simulink model "full_state_linear_SPMSG"  (R2020b)
settings: Solver=FixedStepAuto  StartTime=0  StopTime=2  FixedStep=5e-7  RelTol=1e-3
undefined symbols (not defined in the file): capacitance, DiscIntNeverNeededParam, LdRated, LqRated, PhiPMRated, Pn, Rsnubber, RsRated, speed, TsimCurLoop, TsimMotor
libraries: powerlib x18, slpidlib x3, simulink x2, powerlib_meascontrol x2
(part 1 of 2)
settings Model: SimulationMode=accelerator  Creator=73775  LastModifiedBy=73775
settings DataIOCC: ReturnWorkspaceOutputs=off

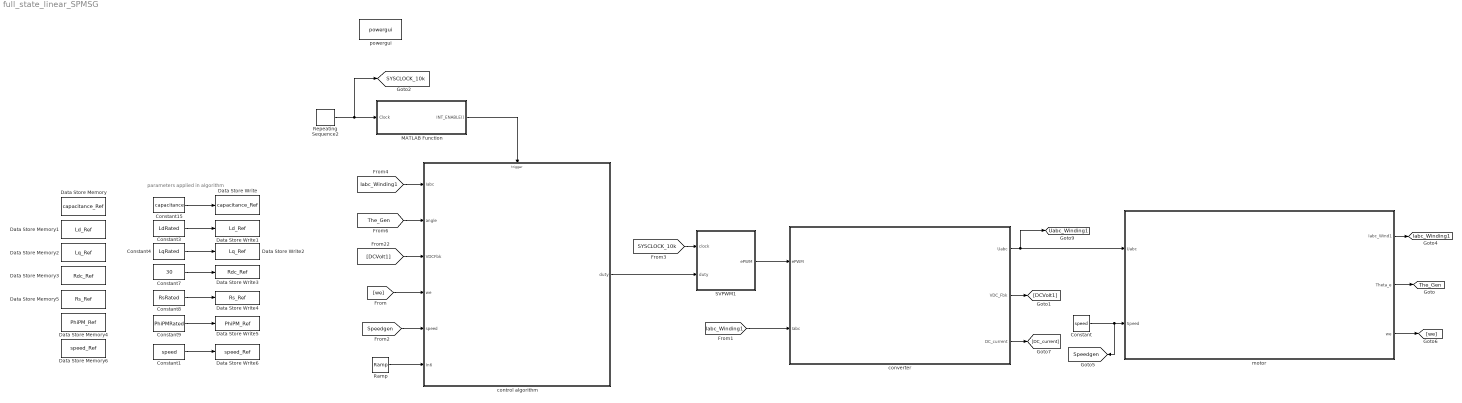
== system full_state_linear_SPMSG ==
  note: parameters applied in algorithm
  Constant : Constant  Value=speed  SampleTime=TsimMotor
  Constant1 : Constant  Value=speed  SampleTime=TsimMotor
  Constant15 : Constant  Value=capacitance  SampleTime=TsimMotor
  Constant3 : Constant  Value=LdRated  SampleTime=TsimMotor
  Constant4 : Constant  Value=LqRated  SampleTime=TsimMotor
  Constant7 : Constant  Value=30  SampleTime=TsimMotor
  Constant8 : Constant  Value=RsRated  SampleTime=TsimMotor
  Constant9 : Constant  Value=PhiPMRated  SampleTime=TsimMotor
  Data Store Memory : DataStoreMemory  DataStoreName=capacitance_Ref  ReadBeforeWriteMsg=warning  WriteAfterWriteMsg=warning  WriteAfterReadMsg=warning  ShowAdditionalParam=off
  Data Store Memory1 : DataStoreMemory  DataStoreName=Ld_Ref  ReadBeforeWriteMsg=warning  WriteAfterWriteMsg=warning  WriteAfterReadMsg=warning  ShowAdditionalParam=off
  Data Store Memory2 : DataStoreMemory  DataStoreName=Lq_Ref  ReadBeforeWriteMsg=warning  WriteAfterWriteMsg=warning  WriteAfterReadMsg=warning  ShowAdditionalParam=off
  Data Store Memory3 : DataStoreMemory  DataStoreName=Rdc_Ref  ReadBeforeWriteMsg=warning  WriteAfterWriteMsg=warning  WriteAfterReadMsg=warning  ShowAdditionalParam=off
  Data Store Memory4 : DataStoreMemory  DataStoreName=PhiPM_Ref  ReadBeforeWriteMsg=warning  WriteAfterWriteMsg=warning  WriteAfterReadMsg=warning  ShowAdditionalParam=off
  Data Store Memory5 : DataStoreMemory  DataStoreName=Rs_Ref  ReadBeforeWriteMsg=warning  WriteAfterWriteMsg=warning  WriteAfterReadMsg=warning  ShowAdditionalParam=off
  Data Store Memory6 : DataStoreMemory  DataStoreName=speed_Ref  ReadBeforeWriteMsg=warning  WriteAfterWriteMsg=warning  WriteAfterReadMsg=warning  ShowAdditionalParam=off
  Data Store Write : DataStoreWrite  DataStoreName=capacitance_Ref
  Data Store Write1 : DataStoreWrite  DataStoreName=Ld_Ref
  Data Store Write2 : DataStoreWrite  DataStoreName=Lq_Ref
  Data Store Write3 : DataStoreWrite  DataStoreName=Rdc_Ref
  Data Store Write4 : DataStoreWrite  DataStoreName=Rs_Ref
  Data Store Write5 : DataStoreWrite  DataStoreName=PhiPM_Ref
  Data Store Write6 : DataStoreWrite  DataStoreName=speed_Ref
  MATLAB Function : MATLAB Function  TreatAsAtomicUnit=on
  Ramp : simulink/Sources/Ramp  slope=1000  start=0  InitialOutput=28
  Repeating Sequence2 : simulink/Sources/Repeating Sequence  rep_seq_t=[0 0.5*TsimCurLoop 1*TsimCurLoop]  rep_seq_y=[0 1/20000 0]
  SVPWM1 : Subsystem
  control algorithm : Subsystem  TreatAsAtomicUnit=on
  converter : Subsystem
  motor : Subsystem
  powergui : powerlib/powergui  Priority=1  SimulationMode=Discrete  SampleTime=TsimMotor  frequency=60  Iterations=50  frequencyindice=0  Pbase=100e6  ErrMax=1e-4  UnitsV=kV  UnitsW=MW  buscounter=0  FunctionMessages=off  echomessages=off  EnableUseOfTLC=off  CurrentSourceSwitches=off  DisableSnubberDevices=off  DisableRonSwitches=off  DisableVfSwitches=off  DisplayEquations=off  AutomaticDiscreteSolvers=off  SolverType=Tustin/Backward Euler (TBE)  Interpol=off  ExternalGateDelay=off  methode=off  Ts=100  x0status=blocks  SPID=on  SwTol=0  HookPort=off  NonlinearTolerance=1e-4  nMaxIteration=100  ContinueOnMaxIteration=off  RestoreLinks=warning  ResistiveCurrentMeasurement=off  Frange=[0:2:500]  Ylog=off  Xlog=on  ShowGrid=off  save=off  variable=ZData  structure=Ia  ZoomFFT=off  StartTime=0.2  cycles=5  DisplayStyle=3  fundamental=67  FreqAxis=on  MaxFrequency=2000  frequencyindicesteady=1  RmsSteady=1  display=off
  tag scope: Iabc_Winding1=global, SYSCLOCK_10k=global, Speedgen=global, The_Gen=global, Uabc_Winding1=global
  wires:
  motor/2(Theta_e) -> [The_Gen]
  motor/1(Iabc_Wind1) -> [Iabc_Winding1]
  MATLAB Function/1(INT_ENABLE()) -> control algorithm/Trigger
  Repeating Sequence2/1 -> [SYSCLOCK_10k], MATLAB Function/1(Clock)
  control algorithm/1(duty) -> SVPWM1/2(duty)
  [SYSCLOCK_10k] -> SVPWM1/1(clock)
  motor/3(we) -> [we]
  [we] -> control algorithm/4(we)
  Constant/1 -> [Speedgen], motor/2("Speed ")
  [The_Gen] -> control algorithm/2(angle)
  [Speedgen] -> control algorithm/5(speed)
  converter/1(Uabc) -> [Uabc_Winding1], motor/1(Uabc)
  SVPWM1/1(ePWM) -> converter/1(ePWM)
  [Iabc_Winding1] -> converter/2(Iabc)
  converter/2(VDC_Fbk) -> [DCVolt1]
  converter/3(DC_current) -> [DC_current]
  [Iabc_Winding1] -> control algorithm/1(Iabc)
  [DCVolt1] -> control algorithm/3(VDCFbk)
  Ramp/1 -> control algorithm/6(In6)
  Constant15/1 -> Data Store Write/1
  Constant3/1 -> Data Store Write1/1
  Constant4/1 -> Data Store Write2/1
  Constant7/1 -> Data Store Write3/1
  Constant8/1 -> Data Store Write4/1
  Constant9/1 -> Data Store Write5/1
  Constant1/1 -> Data Store Write6/1

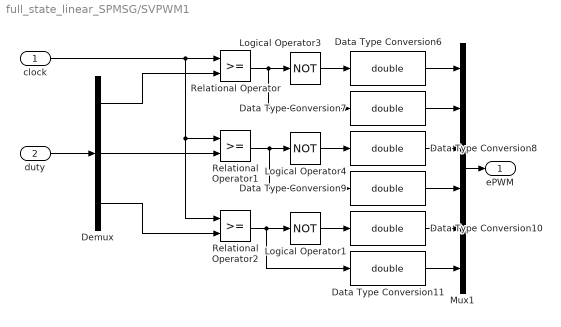
== system full_state_linear_SPMSG/SVPWM1 ==
  clock : Inport
  duty : Inport  Port=2
  Data Type Conversion{6..11} (6 alike) : DataTypeConversion  OutDataTypeStr=double
  Demux : Demux  Outputs=3
  Logical Operator1 : Logic  Operator=NOT  AllPortsSameDT=off  OutDataTypeStr=boolean
  Logical Operator3 : Logic  Operator=NOT  AllPortsSameDT=off  OutDataTypeStr=boolean
  Logical Operator4 : Logic  Operator=NOT  AllPortsSameDT=off  OutDataTypeStr=boolean
  Mux1 : Mux  Inputs=6
  Relational Operator : RelationalOperator  OutDataTypeStr=boolean  RndMeth=Simplest
  Relational Operator1 : RelationalOperator  OutDataTypeStr=boolean  RndMeth=Simplest
  Relational Operator2 : RelationalOperator  OutDataTypeStr=boolean  RndMeth=Simplest
  ePWM : Outport
  wires:
  Data Type Conversion6/1 -> Mux1/1
  Data Type Conversion11/1 -> Mux1/6
  Data Type Conversion7/1 -> Mux1/2
  Data Type Conversion10/1 -> Mux1/5
  Data Type Conversion9/1 -> Mux1/4
  Data Type Conversion8/1 -> Mux1/3
  duty/1 -> Demux/1
  Demux/3 -> Relational Operator2/2
  Mux1/1 -> ePWM/1
  Demux/2 -> Relational Operator1/2
  Relational Operator/1 -> Data Type Conversion7/1, Logical Operator3/1
  Demux/1 -> Relational Operator/2
  Relational Operator2/1 -> Data Type Conversion11/1, Logical Operator1/1
  clock/1 -> Relational Operator/1, Relational Operator1/1, Relational Operator2/1
  Relational Operator1/1 -> Data Type Conversion9/1, Logical Operator4/1
  Logical Operator3/1 -> Data Type Conversion6/1
  Logical Operator4/1 -> Data Type Conversion8/1
  Logical Operator1/1 -> Data Type Conversion10/1

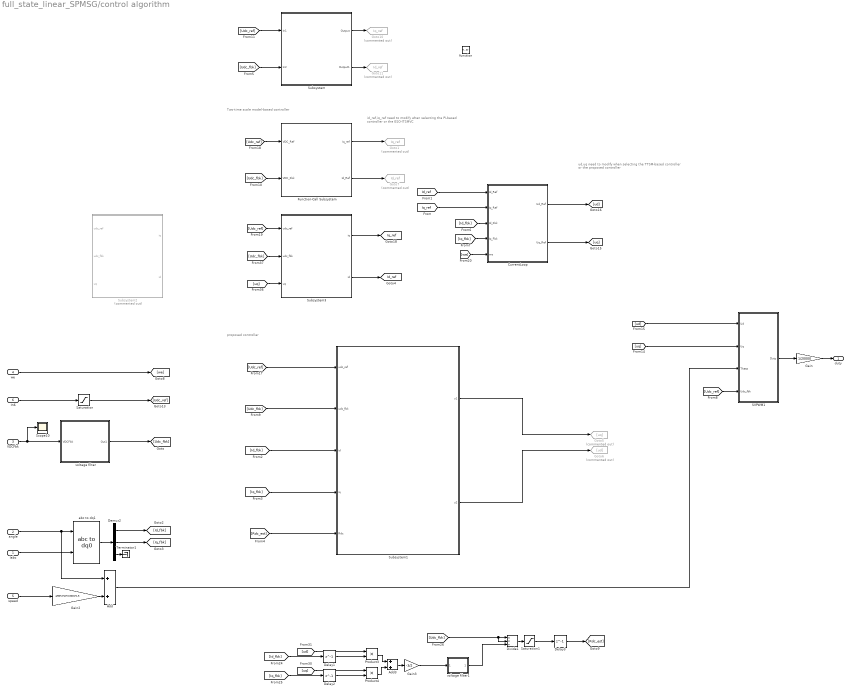
== system full_state_linear_SPMSG/control algorithm ==
  note: proposed controller
  note: Two-time scale model-based controller
  note: ud,uq
      | need to modify when selecting the TTSM-based
      | controller or the proposed controller
  note: id_ref,iq_ref
      | need to modify when selecting the PI-based
      | controller or the ESO-ITSMVC
  Iabc : Inport
  angle : Inport  Port=2
  VDCFbk : Inport  Port=3
  we : Inport  Port=4
  speed : Inport  Port=5
  In6 : Inport  Port=6
  function : TriggerPort  TriggerType=function-call  VariantControl=Variant
  Add : Sum
  Add3 : Sum
  CurrentLoop : Subsystem  mask{kp=0.075, ki=100}
      mask Display:
      | color('blue');
      | disp('current controller');
      | color('black');
      | port_label('input',1,'Id ref','texmode','on');
      | port_label('input',2,'Iq ref','texmode','on');
      | port_label('input',3,'Id fbk','texmode','on');
      | port_label('input',4,'Iq fbk','texmode','on');
      | port_label('input',5,'we','texmode','on');
      | port_label('output',1,'ud ref','texmode','on');
      | port_label('output',2,'uq ref','texmode','on');
  Delay1 : Delay  DelayLength=1
  Delay2 : Delay  DelayLength=1
  Delay3 : Delay  DelayLength=1
  Demux2 : Demux  Outputs=3
  Divide1 : Product  Inputs=**/
  Function-Call Subsystem : Subsystem  TreatAsAtomicUnit=on  mask{kp=0.03, ki=1.6}
      mask Display:
      | color('blue');
      | disp('PI-based voltage controller');
      | color('black');
      | port_label('input',1,'Udc ref','texmode','on');
      | port_label('input',2,'Udc fbk','texmode','on');
      | port_label('output',1,'Iq ref','texmode','on');
      | port_label('output',2,'Id ref','texmode','on');
  Gain : Gain  Gain=1/20000
  Gain2 : Gain  Gain=4/60*2*pi*0.0001*1.5
  Gain3 : Gain  Gain=-3/2
  Goto1 : Goto  Commented=on  GotoTag=Iq_ref  TagVisibility=global
  Goto10 : Goto  Commented=on  GotoTag=Iq_ref  TagVisibility=global
  Goto11 : Goto  Commented=on  GotoTag=Id_ref  TagVisibility=global
  Goto5 : Goto  Commented=on  GotoTag=uq
  Goto6 : Goto  Commented=on  GotoTag=ud
  Goto7 : Goto  Commented=on  GotoTag=Id_ref  TagVisibility=global
  Product3 : Product
  Product4 : Product
  SVPWM1 : Subsystem
  Saturation : Saturate  UpperLimit=48  LowerLimit=0
  Saturation1 : Saturate  UpperLimit=100  LowerLimit=10
  Scope10 : Scope
  Subsystem : Subsystem  mask{k=0.06, n=1e-3}
      mask Display:
      | color('blue');
      | disp('adaptive voltage controller');
      | color('black');
      | port_label('input',1,'Udc ref','texmode','on');
      | port_label('input',2,'Udc fbk','texmode','on');
      | port_label('output',1,'Iq ref','texmode','on');
      | port_label('output',2,'Id ref','texmode','on');
  Subsystem1 : Subsystem  mask{k0=235000000, k1=11990000, k2=5000, k3=800, k4=160000, k5=0.15}
      mask Display:
      | color('blue');
      | disp('proposed integrated controller');
      | color('black');
      | port_label('input',1,'Udc ref','texmode','on');
      | port_label('input',2,'Udc fbk','texmode','on');
      | port_label('input',3,'Id fbk','texmode','on');
      | port_label('input',4,'Iq fbk','texmode','on');
      | port_label('output',1,'uq','texmode','on');
      | port_label('output',2,'ud','texmode','on');
  Subsystem2 : Subsystem  Commented=on  mask{c=0.1, r=0.017, n=0.02, b1=170, b2=14500}
      mask prompts: c "intergrel term in s"; r "product term of s"; n "product term of sgn(s)"; b1 "b1 in ESO"; b2 "b2 in ESO"
      mask Display:
      | color('blue');
      | disp('ESO-ITSMVC');
      | color('black');
      | port_label('input',1,'Udc ref','texmode','on');
      | port_label('input',2,'Udc fbk','texmode','on');
      | port_label('input',3,'uq','texmode','on');
      | port_label('output',1,'Iq ref','texmode','on');
      | port_label('output',2,'Id ref','texmode','on');
  Subsystem3 : Subsystem  mask{c=250, r=0.06, n=0.02, b1=3000, b2=2250000}
      mask prompts: c "intergrel term in s"; r "product term of s"; n "product term of sgn(s)"; b1 "b1 in ESO"; b2 "b2 in ESO"
      mask Display:
      | color('blue');
      | disp('ESO-ITSMVC');
      | color('black');
      | port_label('input',1,'Udc ref','texmode','on');
      | port_label('input',2,'Udc fbk','texmode','on');
      | port_label('input',3,'uq','texmode','on');
      | port_label('output',1,'Iq ref','texmode','on');
      | port_label('output',2,'Id ref','texmode','on');
  Terminator1 : Terminator
  abc to dq1 : powerlib_meascontrol/Transformations/abc to dq0  Alignment=Aligned with phase A axis
  voltage filter : Subsystem
  voltage filter1 : Subsystem
  duty : Outport
  tag scope: Id_ref=global, Iq_ref=global
  wires:
  Iabc/1 -> abc to dq1/1
  abc to dq1/1 -> Demux2/1
  Demux2/3 -> Terminator1/1
  [Id_ref] -> CurrentLoop/1(Id_Ref)
  [Iq_ref] -> CurrentLoop/2(Iq_Ref)
  Demux2/1 -> [Id_fbk]
  Demux2/2 -> [Iq_fbk]
  we/1 -> [we]
  SVPWM1/1(Duty) -> Gain/1
  Gain/1 -> duty/1
  VDCFbk/1 -> voltage filter/1(VDCFbk), Scope10/1
  Add/1 -> SVPWM1/3(Theta)
  speed/1 -> Gain2/1
  Gain2/1 -> Add/2
  [Udc_ref] -> SVPWM1/4(Udc_fbk)
  CurrentLoop/1(Ud_Ref) -> [ud]
  CurrentLoop/2(Uq_Ref) -> [uq]
  angle/1 -> Add/1, abc to dq1/2
  [ud] -> SVPWM1/1(Ud)
  [uq] -> SVPWM1/2(Uq)
  [Udc_ref] -> Function-Call Subsystem/1(VDC_Ref)
  [Udc_fbk] -> Function-Call Subsystem/2(VDC_Fbk)
  In6/1 -> Saturation/1
  [uq] -> Subsystem3/3(uq)
  [Id_fbk] -> CurrentLoop/3(Id_Fbk)
  [Iq_fbk] -> CurrentLoop/4(Iq_Fbk)
  Saturation/1 -> [Udc_ref]
  Subsystem3/1(iq) -> [Iq_ref]
  Subsystem3/2(id) -> [Id_ref]
  [Udc_ref] -> Subsystem3/1(udc_ref)
  [Udc_fbk] -> Subsystem3/2(udc_fbk)
  [we] -> CurrentLoop/5(we)
  [Udc_ref] -> Subsystem1/1(udc_ref)
  [Udc_fbk] -> Subsystem1/2(udc_fbk)
  Subsystem1/1(u1) -> Goto5/1
  Subsystem1/2(u2) -> Goto6/1
  [Id_fbk] -> Subsystem1/3(id)
  [Iq_fbk] -> Subsystem1/4(iq)
  Function-Call Subsystem/2(Id_Ref) -> Goto7/1
  voltage filter/1(Out1) -> [Udc_fbk]
  Product3/1 -> Add3/1
  Add3/1 -> Gain3/1
  [ud] -> Product3/1
  Delay1/1 -> Product3/2
  Divide1/1 -> Saturation1/1
  [uq] -> Product4/1
  Product4/1 -> Add3/2
  [Udc_fbk] -> Divide1/1, Divide1/2
  [Id_fbk] -> Delay1/1
  Delay2/1 -> Product4/2
  [Iq_fbk] -> Delay2/1
  [Rdc_est] -> Subsystem1/5(Rdc)
  Saturation1/1 -> Delay3/1
  Gain3/1 -> voltage filter1/1(VDCFbk)
  voltage filter1/1(Out1) -> Divide1/3
  Delay3/1 -> [Rdc_est]
  [Udc_ref] -> Subsystem/1(In1)
  [Udc_fbk] -> Subsystem/2(In2)
  Subsystem/1(Output) -> Goto10/1
  Subsystem/2(Output1) -> Goto11/1
  Function-Call Subsystem/1(Iq_ref) -> Goto1/1

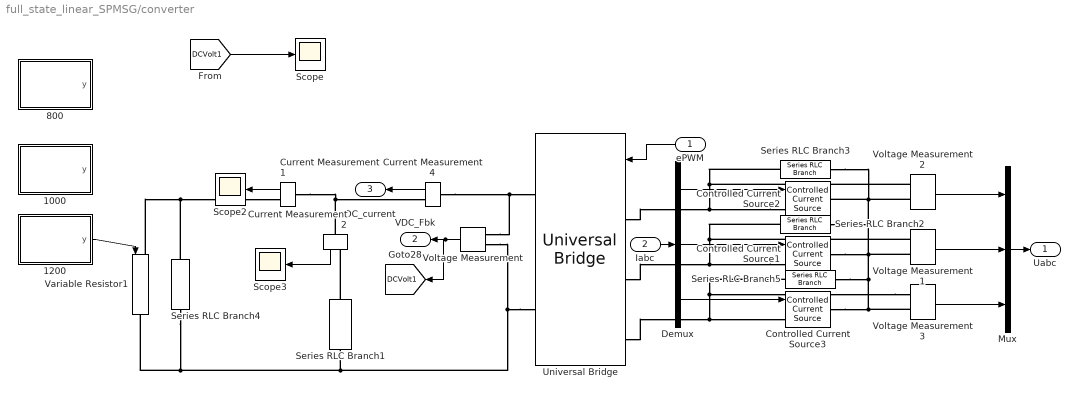
== system full_state_linear_SPMSG/converter ==
  ePWM : Inport
  Iabc : Inport  Port=2
  1000 : MATLAB Function  TreatAsAtomicUnit=on
  1200 : MATLAB Function  TreatAsAtomicUnit=on
  800 : MATLAB Function  TreatAsAtomicUnit=on
  Controlled Current Source1 : powerlib/Electrical Sources/Controlled Current Source  Initialize=on  Source_Type=AC  Amplitude=0  Phase=0  Frequency=0  Measurements=None
  Controlled Current Source2 : powerlib/Electrical Sources/Controlled Current Source  Initialize=on  Source_Type=AC  Amplitude=0  Phase=0  Frequency=0  Measurements=None
  Controlled Current Source3 : powerlib/Electrical Sources/Controlled Current Source  Initialize=on  Source_Type=AC  Amplitude=0  Phase=0  Frequency=0  Measurements=None
  Current Measurement1 : powerlib/Measurements/Current Measurement  PhasorSimulation=off  OutputType=Complex  PSBequivalent=0
  Current Measurement2 : powerlib/Measurements/Current Measurement  PhasorSimulation=off  OutputType=Complex  PSBequivalent=0
  Current Measurement4 : powerlib/Measurements/Current Measurement  PhasorSimulation=off  OutputType=Complex  PSBequivalent=0
  Demux : Demux  Outputs=3
  Mux : Mux  Inputs=3
  Scope : Scope
  Scope2 : Scope
  Scope3 : Scope
  Series RLC Branch1 : powerlib/Elements/Series RLC Branch  LConnTagsString=__new0  RConnTagsString=__new0  BranchType=C  Resistance=1  Inductance=51.869e-9  SetiL0=off  InitialCurrent=0  Capacitance=capacitance  Setx0=on  InitialVoltage=28  Measurements=None
  Series RLC Branch2 : powerlib/Elements/Series RLC Branch  LConnTagsString=__new0  RConnTagsString=__new0  BranchType=R  Resistance=Rsnubber  Inductance=51.869e-9  SetiL0=off  InitialCurrent=0  Capacitance=330e-6  Setx0=off  InitialVoltage=0  Measurements=None
  Series RLC Branch3 : powerlib/Elements/Series RLC Branch  LConnTagsString=__new0  RConnTagsString=__new0  BranchType=R  Resistance=Rsnubber  Inductance=51.869e-9  SetiL0=off  InitialCurrent=0  Capacitance=330e-6  Setx0=off  InitialVoltage=0  Measurements=None
  Series RLC Branch4 : powerlib/Elements/Series RLC Branch  LConnTagsString=__new0  RConnTagsString=__new0  BranchType=R  Resistance=100  Inductance=51.869e-9  SetiL0=off  InitialCurrent=0  Capacitance=330e-6  Setx0=off  InitialVoltage=0  Measurements=None
  Series RLC Branch5 : powerlib/Elements/Series RLC Branch  LConnTagsString=__new0  RConnTagsString=__new0  BranchType=R  Resistance=Rsnubber  Inductance=51.869e-9  SetiL0=off  InitialCurrent=0  Capacitance=330e-6  Setx0=off  InitialVoltage=0  Measurements=None
  Universal Bridge : powerlib/Power Electronics/Universal Bridge  Arms=3  SnubberResistance=Rsnubber  SnubberCapacitance=inf  Device=IGBT / Diodes  Ron=0.02  Lon=0  ForwardVoltages="[  0  0  ]"  ForwardVoltage=0  GTOparameters=[ 10e-6 , 20e-6 ]  IGBTparameters=[ 1e-6 , 2e-6 ]  Measurements=None  Measurements_2=None  converterType=Rectifier
  Variable Resistor1 : powerlib/Elements/Variable Resistor  Rabsmin=1e-3
      settings: SourceProductBaseCode=PS
  Voltage Measurement{,1..3} (4 alike) : powerlib/Measurements/Voltage Measurement  PhasorSimulation=off  OutputType=Complex  PSBequivalent=0
  Uabc : Outport
  VDC_Fbk : Outport  Port=2
  DC_current : Outport  Port=3
  tag scope: DCVolt1=global
  wires:
  Voltage Measurement/1 -> [DCVolt1], VDC_Fbk/1
  Demux/1 -> Controlled Current Source2/1
  Demux/3 -> Controlled Current Source3/1
  Voltage Measurement1/1 -> Mux/2
  Voltage Measurement2/1 -> Mux/1
  Demux/2 -> Controlled Current Source1/1
  Voltage Measurement3/1 -> Mux/3
  Mux/1 -> Uabc/1
  ePWM/1 -> Universal Bridge/1
  Iabc/1 -> Demux/1
  Current Measurement4/1 -> DC_current/1
  Current Measurement1/1 -> Scope2/1
  Current Measurement2/1 -> Scope3/1
  [DCVolt1] -> Scope/1
  1200/1(y) -> Variable Resistor1/1
  connections:
  Universal Bridge/RConn2 -- Series RLC Branch4/RConn1 -- Variable Resistor1/RConn1 -- Series RLC Branch1/RConn1 -- Voltage Measurement/LConn2
  Voltage Measurement2/LConn2 -- Controlled Current Source2/RConn1 -- Controlled Current Source1/RConn1 -- Voltage Measurement1/LConn2 -- Voltage Measurement3/LConn2 -- Controlled Current Source3/RConn1 -- Series RLC Branch5/RConn1 -- Series RLC Branch2/RConn1 -- Series RLC Branch3/RConn1
  Voltage Measurement/LConn1 -- Current Measurement4/LConn1 -- Universal Bridge/RConn1
  Controlled Current Source2/LConn1 -- Universal Bridge/LConn1 -- Voltage Measurement2/LConn1 -- Series RLC Branch3/LConn1
  Voltage Measurement3/LConn1 -- Controlled Current Source3/LConn1 -- Universal Bridge/LConn3 -- Series RLC Branch5/LConn1
  Controlled Current Source1/LConn1 -- Universal Bridge/LConn2 -- Series RLC Branch2/LConn1 -- Voltage Measurement1/LConn1
  Current Measurement1/LConn1 -- Current Measurement2/LConn1 -- Current Measurement4/RConn1
  Variable Resistor1/LConn1 -- Series RLC Branch4/LConn1 -- Current Measurement1/RConn1
  Series RLC Branch1/LConn1 -- Current Measurement2/RConn1

== system full_state_linear_SPMSG/motor ==
  Uabc : Inport
  "Speed " : Inport  Port=2
  Add : Sum  Inputs=+-
  Clark Transformation : Subsystem
  Demux : Demux  Outputs=3
  Electrical Model Simplied1 : Subsystem
  "Mechanical Model " : Subsystem
  Mux1 : Mux  Inputs=3
  Park Transformation : Subsystem
  VSINonlinearity : Subsystem
  dq0 to abc1 : powerlib_meascontrol/Transformations/dq0 to abc  Alignment=Aligned with phase A axis
  Iabc_Wind1 : Outport
  Theta_e : Outport  Port=2
  we : Outport  Port=3
  wires:
  Clark Transformation/1(Alpha) -> Park Transformation/1(Alpha)
  Clark Transformation/2(Beta) -> Park Transformation/2(Beta)
  "Mechanical Model "/1(Theta_e) -> Park Transformation/3(theta), Theta_e/1, dq0 to abc1/2
  Demux/1 -> Clark Transformation/1(U)
  Demux/2 -> Clark Transformation/2(V)
  Demux/3 -> Clark Transformation/3(W)
  Mux1/1 -> dq0 to abc1/1
  "Mechanical Model "/2(we) -> Electrical Model Simplied1/3(we), we/1
  "Speed "/1 -> "Mechanical Model "/1(speed)
  dq0 to abc1/1 -> VSINonlinearity/1(IABC), Iabc_Wind1/1
  Park Transformation/1(D) -> Electrical Model Simplied1/1(Ud)
  Park Transformation/2(Q) -> Electrical Model Simplied1/2(Uq)
  Electrical Model Simplied1/1(Id) -> Mux1/1
  Electrical Model Simplied1/2(Iq) -> Mux1/2
  Add/1 -> Demux/1
  Uabc/1 -> Add/1
  VSINonlinearity/1(UError) -> Add/2

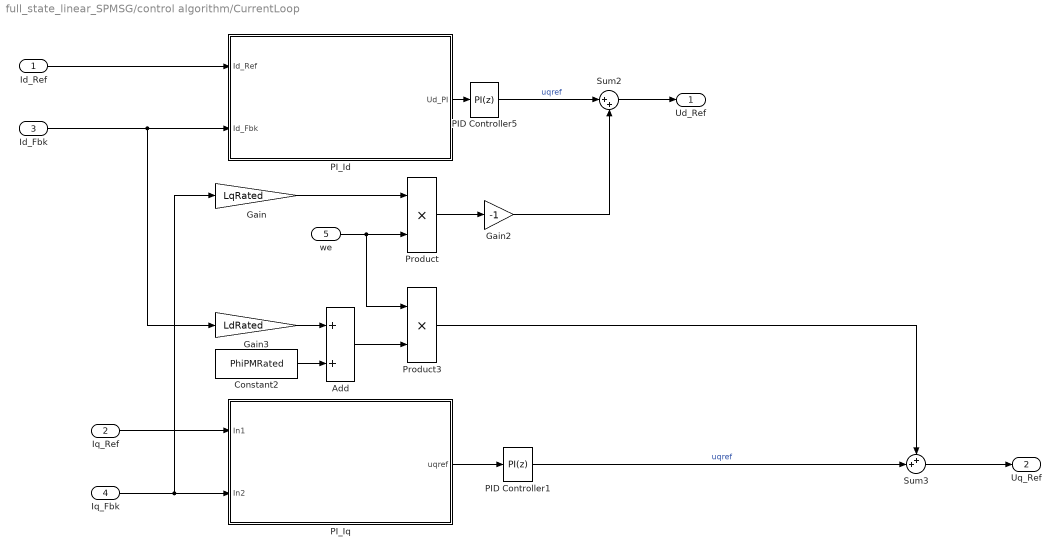
== system full_state_linear_SPMSG/control algorithm/CurrentLoop ==
  Id_Ref : Inport
  Iq_Ref : Inport  Port=2
  Id_Fbk : Inport  Port=3
  Iq_Fbk : Inport  Port=4
  we : Inport  Port=5
  Add : Sum
  Constant2 : Constant  Value=PhiPMRated  SampleTime=-1
  Gain : Gain  Gain=LqRated
  Gain2 : Gain  Gain=-1
  Gain3 : Gain  Gain=LdRated
  PID Controller1 : slpidlib/PID Controller  Controller=PI  Form=Parallel  TimeDomain=Discrete-time  UseExternalTs=off  SampleTime=-1  IntegratorMethod=Forward Euler  FilterMethod=Forward Euler  ControllerParametersSource=internal  P=kp  I=ki  D=0  UseFilter=on  N=100  TunerSelectOption=Transfer Function Based (PID Tuner App)  InitialConditionSource=internal  InitialConditionForIntegrator=0  InitialConditionForFilter=0  DifferentiatorICPrevScaledInput=0  ExternalReset=none  TrackingMode=off  Kt=1  LimitOutput=on  SatLimitsSource=internal  UpperSaturationLimit=800  LowerSaturationLimit=-800  LinearizeAsGain=on  AntiWindupMode=none  Kb=1  POutMin=[]  POutMax=[]  IOutMin=[]  IOutMax=[]  DOutMin=[]  DOutMax=[]  NOutMin=[]  NOutMax=[]  SumOutMin=-800  SumOutMax=800  SaturationOutMin=-800  SaturationOutMax=800  PParamMin=[]  PParamMax=[]  IParamMin=[]  IParamMax=[]  DParamMin=[]  DParamMax=[]  NParamMin=[]  NParamMax=[]  KbParamMin=[]  KbParamMax=[]  KtParamMin=[]  KtParamMax=[]  KbOutMin=[]  KbOutMax=[]  KtOutMin=[]  KtOutMax=[]  IntegratorOutMin=[]  IntegratorOutMax=[]  FilterOutMin=[]  FilterOutMax=[]  SumI1OutMin=[]  SumI1OutMax=[]  SumI2OutMin=[]  SumI2OutMax=[]  SumI3OutMin=[]  SumI3OutMax=[]  SumI4OutMin=[]  SumI4OutMax=[]  SumDOutMin=[]  SumDOutMax=[]  DifferentiatorOutMin=[]  DifferentiatorOutMax=[]  FilterDiffOutCoefMin=[]  FilterDiffOutCoefMax=[]  ReciprocalOutMin=[]  ReciprocalOutMax=[]  SumDenOutMin=[]  SumDenOutMax=[]  SumNumOutMin=[]  SumNumOutMax=[]  DivideOutMin=[]  DivideOutMax=[]  UdiffTsProdOutMin=[]  UdiffTsProdOutMax=[]  NTsProdOutMin=[]  NTsProdOutMax=[]  UintegralTsProdOutMin=[]  UintegralTsProdOutMax=[]  UngainTsProdOutMin=[]  UngainTsProdOutMax=[]  IntegratorContinuousStateAttributes=''  IntegratorStateMustResolveToSignalObject=off  IntegratorRTWStateStorageClass=Auto  FilterContinuousStateAttributes=''  FilterStateMustResolveToSignalObject=off  FilterRTWStateStorageClass=Auto  ParallelPVariant=InternalParameters  IdealPVariant=Disabled  IVariant=InternalParameters  DVariant=Disabled  IntegratorVariant=Discrete  SatVariant=Enabled  AWVariant=Passthrough  PCopyVariant=Disabled  TRVariant=Disabled  FdbkBlocksVariant=Forward  IdealPFdbkVariant=Disabled  SatFdbkVariant=Disabled  DerivativeFilterVariant=Disabled  NVariant=Disabled  NCopyVariant=Disabled_SignalSpec  FilterICVariant=Disabled  IntegratorICVariant=InternalICs  ExternalResetVariant=Disabled  TRSumVariant=Passthrough  SumFdbkVariant=Disabled  SumVariant=Sum_PI  TsampFilterVariant=InternalTs  TsampNgainVariant=Passthrough  TsampIntegralVariant=Passthrough  ExternalSaturationOutDataTypeStr=Inherit: Same as second input
  PID Controller5 : slpidlib/PID Controller  Controller=PI  Form=Parallel  TimeDomain=Discrete-time  UseExternalTs=off  SampleTime=-1  IntegratorMethod=Forward Euler  FilterMethod=Forward Euler  ControllerParametersSource=internal  P=kp  I=ki  D=0  UseFilter=on  N=100  TunerSelectOption=Transfer Function Based (PID Tuner App)  InitialConditionSource=internal  InitialConditionForIntegrator=0  InitialConditionForFilter=0  DifferentiatorICPrevScaledInput=0  ExternalReset=none  TrackingMode=off  Kt=1  LimitOutput=on  SatLimitsSource=internal  UpperSaturationLimit=800  LowerSaturationLimit=-800  LinearizeAsGain=on  AntiWindupMode=none  Kb=1  POutMin=[]  POutMax=[]  IOutMin=[]  IOutMax=[]  DOutMin=[]  DOutMax=[]  NOutMin=[]  NOutMax=[]  SumOutMin=-800  SumOutMax=800  SaturationOutMin=-800  SaturationOutMax=800  PParamMin=[]  PParamMax=[]  IParamMin=[]  IParamMax=[]  DParamMin=[]  DParamMax=[]  NParamMin=[]  NParamMax=[]  KbParamMin=[]  KbParamMax=[]  KtParamMin=[]  KtParamMax=[]  KbOutMin=[]  KbOutMax=[]  KtOutMin=[]  KtOutMax=[]  IntegratorOutMin=[]  IntegratorOutMax=[]  FilterOutMin=[]  FilterOutMax=[]  SumI1OutMin=[]  SumI1OutMax=[]  SumI2OutMin=[]  SumI2OutMax=[]  SumI3OutMin=[]  SumI3OutMax=[]  SumI4OutMin=[]  SumI4OutMax=[]  SumDOutMin=[]  SumDOutMax=[]  DifferentiatorOutMin=[]  DifferentiatorOutMax=[]  FilterDiffOutCoefMin=[]  FilterDiffOutCoefMax=[]  ReciprocalOutMin=[]  ReciprocalOutMax=[]  SumDenOutMin=[]  SumDenOutMax=[]  SumNumOutMin=[]  SumNumOutMax=[]  DivideOutMin=[]  DivideOutMax=[]  UdiffTsProdOutMin=[]  UdiffTsProdOutMax=[]  NTsProdOutMin=[]  NTsProdOutMax=[]  UintegralTsProdOutMin=[]  UintegralTsProdOutMax=[]  UngainTsProdOutMin=[]  UngainTsProdOutMax=[]  IntegratorContinuousStateAttributes=''  IntegratorStateMustResolveToSignalObject=off  IntegratorRTWStateStorageClass=Auto  FilterContinuousStateAttributes=''  FilterStateMustResolveToSignalObject=off  FilterRTWStateStorageClass=Auto  ParallelPVariant=InternalParameters  IdealPVariant=Disabled  IVariant=InternalParameters  DVariant=Disabled  IntegratorVariant=Discrete  SatVariant=Enabled  AWVariant=Passthrough  PCopyVariant=Disabled  TRVariant=Disabled  FdbkBlocksVariant=Forward  IdealPFdbkVariant=Disabled  SatFdbkVariant=Disabled  DerivativeFilterVariant=Disabled  NVariant=Disabled  NCopyVariant=Disabled_SignalSpec  FilterICVariant=Disabled  IntegratorICVariant=InternalICs  ExternalResetVariant=Disabled  TRSumVariant=Passthrough  SumFdbkVariant=Disabled  SumVariant=Sum_PI  TsampFilterVariant=InternalTs  TsampNgainVariant=Passthrough  TsampIntegralVariant=Passthrough  ExternalSaturationOutDataTypeStr=Inherit: Same as second input
  PI_Id : Subsystem
  PI_Iq : Subsystem
  Product : Product
  Product3 : Product
  Sum2 : Sum  Inputs=|++
  Sum3 : Sum  Inputs=++|
  Ud_Ref : Outport
  Uq_Ref : Outport  Port=2
  wires:
  Id_Fbk/1 -> PI_Id/2(Id_Fbk), Gain3/1
  Iq_Ref/1 -> PI_Iq/1(In1)
  Gain/1 -> Product/1
  Gain3/1 -> Add/1
  Constant2/1 -> Add/2
  Add/1 -> Product3/2
  we/1 -> Product3/1, Product/2
  Iq_Fbk/1 -> Gain/1, PI_Iq/2(In2)
  PI_Id/1(Ud_PI) -> PID Controller5/1
  PI_Iq/1(uqref) -> PID Controller1/1
  Product/1 -> Gain2/1
  Sum2/1 -> Ud_Ref/1
  Gain2/1 -> Sum2/2
  Sum3/1 -> Uq_Ref/1
  PID Controller1/1 -> Sum3/2  "uqref"
  Id_Ref/1 -> PI_Id/1(Id_Ref)
  PID Controller5/1 -> Sum2/1  "uqref"
  Product3/1 -> Sum3/1

== system full_state_linear_SPMSG/control algorithm/Function-Call Subsystem ==
  VDC_Ref : Inport
  VDC_Fbk : Inport  Port=2
  Add3 : Sum  Inputs=|+-
  Constant : Constant  Value=0  SampleTime=-1
  Gain : Gain  Gain=-1
  PID Controller1 : slpidlib/PID Controller  Controller=PI  Form=Parallel  TimeDomain=Discrete-time  UseExternalTs=off  SampleTime=-1  IntegratorMethod=Forward Euler  FilterMethod=Forward Euler  ControllerParametersSource=internal  P=kp  I=ki  D=0  UseFilter=on  N=100  TunerSelectOption=Transfer Function Based (PID Tuner App)  InitialConditionSource=internal  InitialConditionForIntegrator=0  InitialConditionForFilter=0  DifferentiatorICPrevScaledInput=0  ExternalReset=none  TrackingMode=off  Kt=1  LimitOutput=off  SatLimitsSource=internal  UpperSaturationLimit=640000  LowerSaturationLimit=-640000  LinearizeAsGain=on  AntiWindupMode=none  Kb=1  POutMin=[]  POutMax=[]  IOutMin=[]  IOutMax=[]  DOutMin=[]  DOutMax=[]  NOutMin=[]  NOutMax=[]  SumOutMin=-800  SumOutMax=800  SaturationOutMin=-800  SaturationOutMax=800  PParamMin=[]  PParamMax=[]  IParamMin=[]  IParamMax=[]  DParamMin=[]  DParamMax=[]  NParamMin=[]  NParamMax=[]  KbParamMin=[]  KbParamMax=[]  KtParamMin=[]  KtParamMax=[]  KbOutMin=[]  KbOutMax=[]  KtOutMin=[]  KtOutMax=[]  IntegratorOutMin=[]  IntegratorOutMax=[]  FilterOutMin=[]  FilterOutMax=[]  SumI1OutMin=[]  SumI1OutMax=[]  SumI2OutMin=[]  SumI2OutMax=[]  SumI3OutMin=[]  SumI3OutMax=[]  SumI4OutMin=[]  SumI4OutMax=[]  SumDOutMin=[]  SumDOutMax=[]  DifferentiatorOutMin=[]  DifferentiatorOutMax=[]  FilterDiffOutCoefMin=[]  FilterDiffOutCoefMax=[]  ReciprocalOutMin=[]  ReciprocalOutMax=[]  SumDenOutMin=[]  SumDenOutMax=[]  SumNumOutMin=[]  SumNumOutMax=[]  DivideOutMin=[]  DivideOutMax=[]  UdiffTsProdOutMin=[]  UdiffTsProdOutMax=[]  NTsProdOutMin=[]  NTsProdOutMax=[]  UintegralTsProdOutMin=[]  UintegralTsProdOutMax=[]  UngainTsProdOutMin=[]  UngainTsProdOutMax=[]  IntegratorContinuousStateAttributes=''  IntegratorStateMustResolveToSignalObject=off  IntegratorRTWStateStorageClass=Auto  FilterContinuousStateAttributes=''  FilterStateMustResolveToSignalObject=off  FilterRTWStateStorageClass=Auto  ParallelPVariant=InternalParameters  IdealPVariant=Disabled  IVariant=InternalParameters  DVariant=Disabled  IntegratorVariant=Discrete  SatVariant=Disabled  AWVariant=Passthrough  PCopyVariant=Disabled  TRVariant=Disabled  FdbkBlocksVariant=Forward  IdealPFdbkVariant=Disabled  SatFdbkVariant=Disabled  DerivativeFilterVariant=Disabled  NVariant=Disabled  NCopyVariant=Disabled_SignalSpec  FilterICVariant=Disabled  IntegratorICVariant=InternalICs  ExternalResetVariant=Disabled  TRSumVariant=Passthrough  SumFdbkVariant=Disabled  SumVariant=Sum_PI  TsampFilterVariant=InternalTs  TsampNgainVariant=Passthrough  TsampIntegralVariant=Passthrough  ExternalSaturationOutDataTypeStr=Inherit: Same as second input
  Product : Product
  Product1 : Product
  Iq_ref : Outport
  Id_Ref : Outport  Port=2
  wires:
  Add3/1 -> PID Controller1/1
  Constant/1 -> Id_Ref/1
  PID Controller1/1 -> Gain/1
  Gain/1 -> Iq_ref/1
  Product/1 -> Add3/1
  VDC_Ref/1 -> Product/1, Product/2
  VDC_Fbk/1 -> Product1/2, Product1/1
  Product1/1 -> Add3/2

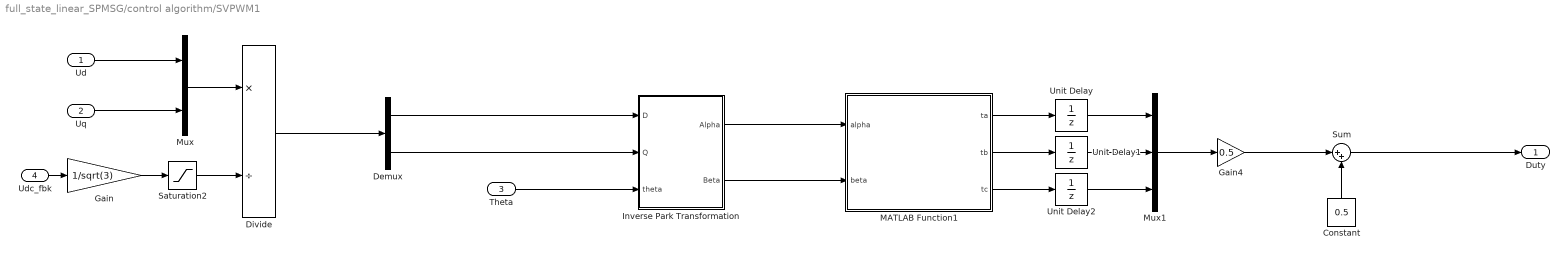
== system full_state_linear_SPMSG/control algorithm/SVPWM1 ==
  Ud : Inport
  Uq : Inport  Port=2
  Theta : Inport  Port=3
  Udc_fbk : Inport  Port=4
  Constant : Constant  Value=0.5  SampleTime=-1
  Demux : Demux  Outputs=2
  Divide : Product  Inputs=*/
  Gain : Gain  Gain=1/sqrt(3)
  Gain4 : Gain  Gain=0.5
  Inverse Park Transformation : Subsystem
  MATLAB Function1 : MATLAB Function  TreatAsAtomicUnit=on
  Mux : Mux  Inputs=2
  Mux1 : Mux  Inputs=3
  Saturation2 : Saturate  UpperLimit=800  LowerLimit=10
  Sum : Sum  Inputs=|++
  Unit Delay : UnitDelay  SampleTime=-1  HasFrameUpgradeWarning=on
  Unit Delay1 : UnitDelay  SampleTime=-1  HasFrameUpgradeWarning=on
  Unit Delay2 : UnitDelay  SampleTime=-1  HasFrameUpgradeWarning=on
  Duty : Outport
  wires:
  Inverse Park Transformation/2(Beta) -> MATLAB Function1/2(beta)
  Divide/1 -> Demux/1
  MATLAB Function1/2(tb) -> Unit Delay1/1
  Mux/1 -> Divide/1
  Saturation2/1 -> Divide/2
  Gain/1 -> Saturation2/1
  Unit Delay1/1 -> Mux1/2
  Inverse Park Transformation/1(Alpha) -> MATLAB Function1/1(alpha)
  Unit Delay2/1 -> Mux1/3
  Theta/1 -> Inverse Park Transformation/3(theta)
  MATLAB Function1/1(ta) -> Unit Delay/1
  MATLAB Function1/3(tc) -> Unit Delay2/1
  Demux/2 -> Inverse Park Transformation/2(Q)
  Demux/1 -> Inverse Park Transformation/1(D)
  Unit Delay/1 -> Mux1/1
  Constant/1 -> Sum/2
  Gain4/1 -> Sum/1
  Mux1/1 -> Gain4/1
  Ud/1 -> Mux/1
  Uq/1 -> Mux/2
  Sum/1 -> Duty/1
  Udc_fbk/1 -> Gain/1

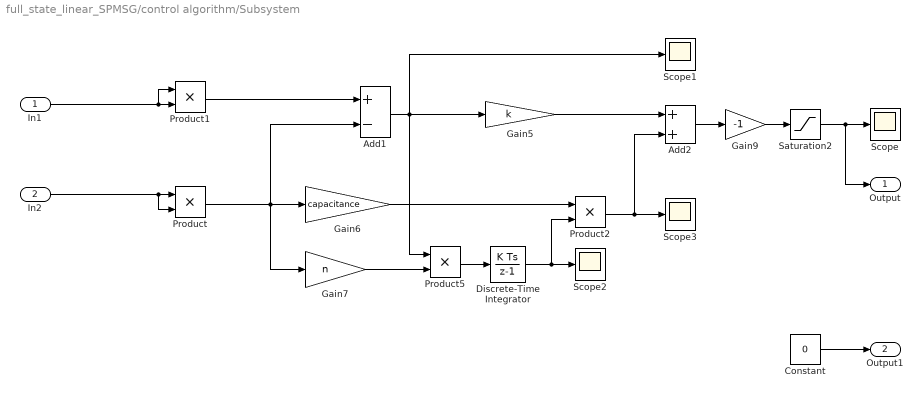
== system full_state_linear_SPMSG/control algorithm/Subsystem ==
  In1 : Inport
  In2 : Inport  Port=2
  Add1 : Sum  Inputs=+-
  Add2 : Sum
  Constant : Constant  Value=0
  Discrete-Time Integrator : DiscreteIntegrator  gainval=1  SampleTime=-1  ICPrevOutput=DiscIntNeverNeededParam  ICPrevScaledInput=DiscIntNeverNeededParam
  Gain5 : Gain  Gain=k
  Gain6 : Gain  Gain=capacitance
  Gain7 : Gain  Gain=n
  Gain9 : Gain  Gain=-1
  Product{,1..2,5} (4 alike) : Product
  Saturation2 : Saturate  UpperLimit=20  LowerLimit=-20
  Scope{,1..3} (4 alike) : Scope
  Output : Outport
  Output1 : Outport  Port=2
  wires:
  Product5/1 -> Discrete-Time Integrator/1
  In2/1 -> Product/2, Product/1
  Add1/1 -> Gain5/1, Scope1/1, Product5/1
  Discrete-Time Integrator/1 -> Product2/2, Scope2/1
  Gain5/1 -> Add2/1
  Gain6/1 -> Product2/1
  Product1/1 -> Add1/1
  Saturation2/1 -> Output/1, Scope/1
  Gain7/1 -> Product5/2
  In1/1 -> Product1/1, Product1/2
  Add2/1 -> Gain9/1
  Product2/1 -> Add2/2, Scope3/1
  Product/1 -> Gain7/1, Add1/2, Gain6/1
  Gain9/1 -> Saturation2/1
  Constant/1 -> Output1/1

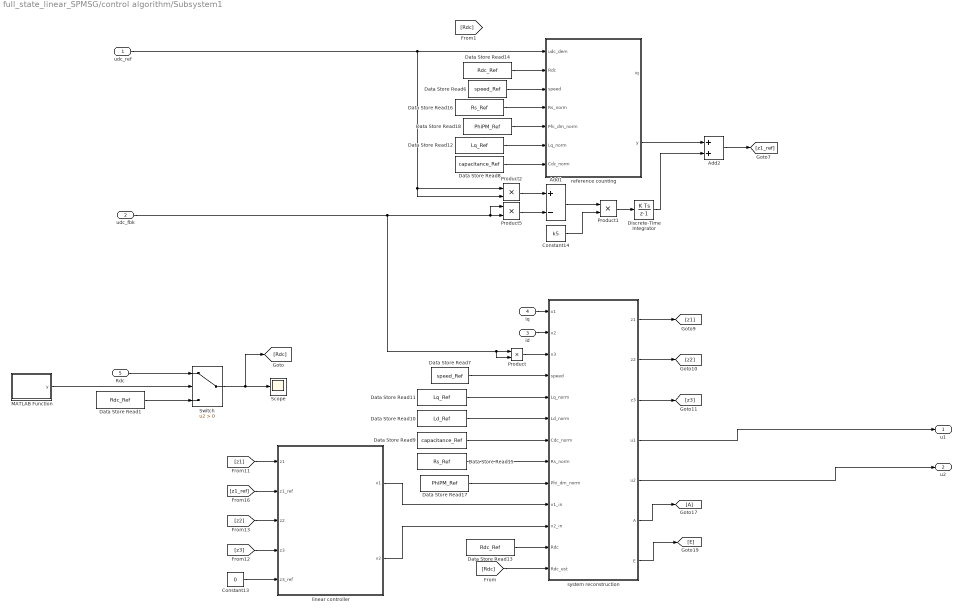
== system full_state_linear_SPMSG/control algorithm/Subsystem1 ==
  udc_ref : Inport
  udc_fbk : Inport  Port=2
  id : Inport  Port=3
  iq : Inport  Port=4
  Rdc : Inport  Port=5
  Add1 : Sum  Inputs=+-
  Add2 : Sum
  Constant13 : Constant  Value=0  SampleTime=-1
  Constant14 : Constant  Value=k5  SampleTime=-1
  Data Store Read1 : DataStoreRead  DataStoreName=Rdc_Ref
  Data Store Read10 : DataStoreRead  DataStoreName=Ld_Ref
  Data Store Read11 : DataStoreRead  DataStoreName=Lq_Ref
  Data Store Read12 : DataStoreRead  DataStoreName=Lq_Ref
  Data Store Read13 : DataStoreRead  DataStoreName=Rdc_Ref
  Data Store Read14 : DataStoreRead  DataStoreName=Rdc_Ref
  Data Store Read15 : DataStoreRead  DataStoreName=Rs_Ref
  Data Store Read16 : DataStoreRead  DataStoreName=Rs_Ref
  Data Store Read17 : DataStoreRead  DataStoreName=PhiPM_Ref
  Data Store Read18 : DataStoreRead  DataStoreName=PhiPM_Ref
  Data Store Read6 : DataStoreRead  DataStoreName=speed_Ref
  Data Store Read7 : DataStoreRead  DataStoreName=speed_Ref
  Data Store Read8 : DataStoreRead  DataStoreName=capacitance_Ref
  Data Store Read9 : DataStoreRead  DataStoreName=capacitance_Ref
  Discrete-Time Integrator : DiscreteIntegrator  SampleTime=-1  ICPrevOutput=DiscIntNeverNeededParam  ICPrevScaledInput=DiscIntNeverNeededParam
  MATLAB Function : MATLAB Function  TreatAsAtomicUnit=on
  Product{,1..2,5} (4 alike) : Product
  Scope : Scope
  Switch : Switch  Criteria=u2 > Threshold
  linear controller : Subsystem
  reference counting : MATLAB Function  TreatAsAtomicUnit=on
  system reconstruction : MATLAB Function  TreatAsAtomicUnit=on
  u1 : Outport
  u2 : Outport  Port=2
  wires:
  Data Store Read11/1 -> system reconstruction/5(Lq_norm)
  [z1] -> linear controller/1(z1)
  system reconstruction/1(z1) -> [z1]
  Data Store Read6/1 -> reference counting/3(speed)
  Data Store Read16/1 -> reference counting/4(Rs_norm)
  Data Store Read8/1 -> reference counting/7(Cdc_norm)
  Data Store Read18/1 -> reference counting/5(Phi_dm_norm)
  Product2/1 -> Add1/1
  [z3] -> linear controller/4(z3)
  Product1/1 -> Discrete-Time Integrator/1
  [z1_ref] -> linear controller/2(z1_ref)
  system reconstruction/7(E) -> [E]
  udc_fbk/1 -> Product/2, Product/1, Product5/1, Product5/2
  system reconstruction/6(A) -> [A]
  Product/1 -> system reconstruction/3(x3)
  Add1/1 -> Product1/1
  Data Store Read7/1 -> system reconstruction/4(speed)
  Constant14/1 -> Product1/2
  Data Store Read9/1 -> system reconstruction/7(Cdc_norm)
  system reconstruction/3(z3) -> [z3]
  Data Store Read15/1 -> system reconstruction/8(Rs_norm)
  linear controller/2(v2) -> system reconstruction/11(v2_in)
  Data Store Read10/1 -> system reconstruction/6(Ld_norm)
  Constant13/1 -> linear controller/5(z3_ref)
  reference counting/2(y) -> Add2/1
  Product5/1 -> Add1/2
  Discrete-Time Integrator/1 -> Add2/2
  linear controller/1(v1) -> system reconstruction/10(v1_in)
  Add2/1 -> [z1_ref]
  Data Store Read12/1 -> reference counting/6(Lq_norm)
  Data Store Read17/1 -> system reconstruction/9(Phi_dm_norm)
  system reconstruction/5(u2) -> u2/1
  system reconstruction/4(u1) -> u1/1
  udc_ref/1 -> Product2/2, Product2/1, reference counting/1(udc_dem)
  id/1 -> system reconstruction/2(x2)
  iq/1 -> system reconstruction/1(x1)
  [z2] -> linear controller/3(z2)
  Switch/1 -> [Rdc], Scope/1
  Data Store Read1/1 -> Switch/3
  Data Store Read14/1 -> reference counting/2(Rdc)
  Data Store Read13/1 -> system reconstruction/12(Rdc)
  [Rdc] -> system reconstruction/13(Rdc_est)
  system reconstruction/2(z2) -> [z2]
  Rdc/1 -> Switch/1
  MATLAB Function/1(y) -> Switch/2

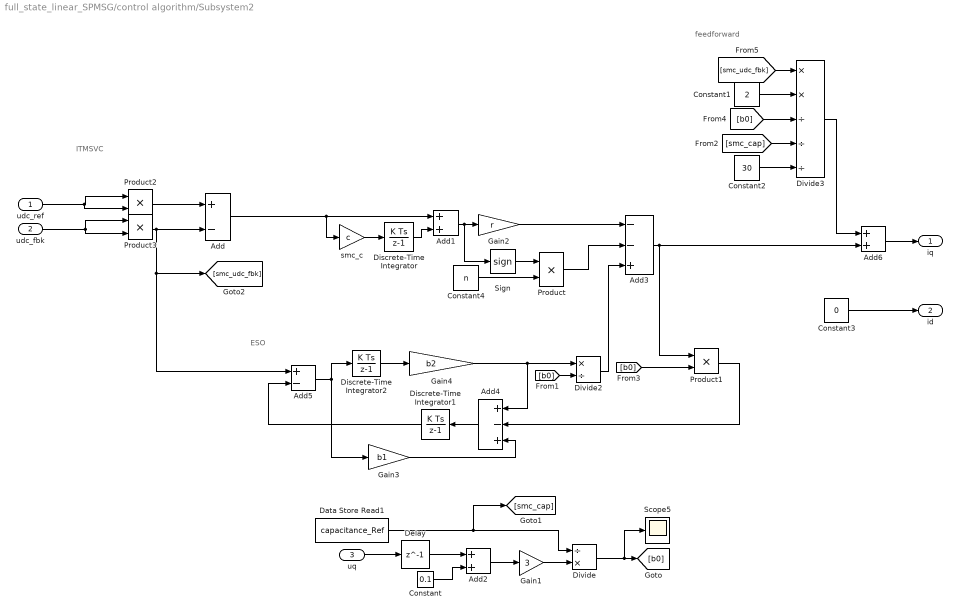
== system full_state_linear_SPMSG/control algorithm/Subsystem2 ==
  note: ESO
  note: feedforward
  note: ITMSVC
  udc_ref : Inport
  udc_fbk : Inport  Port=2
  uq : Inport  Port=3
  Add : Sum  Inputs=+-
  Add1 : Sum
  Add2 : Sum
  Add3 : Sum  Inputs=--+
  Add4 : Sum  Inputs=+-+
  Add5 : Sum  Inputs=+-
  Add6 : Sum
  Constant : Constant  Value=0.1  SampleTime=-1
  Constant1 : Constant  Value=2  SampleTime=-1
  Constant2 : Constant  Value=30  SampleTime=-1
  Constant3 : Constant  Value=0  SampleTime=-1
  Constant4 : Constant  Value=n  SampleTime=-1
  Data Store Read1 : DataStoreRead  DataStoreName=capacitance_Ref
  Delay : Delay  DelayLength=1
  Discrete-Time Integrator : DiscreteIntegrator  SampleTime=-1  ICPrevOutput=DiscIntNeverNeededParam  ICPrevScaledInput=DiscIntNeverNeededParam
  Discrete-Time Integrator1 : DiscreteIntegrator  InitialCondition=2304  SampleTime=-1  ICPrevOutput=DiscIntNeverNeededParam  ICPrevScaledInput=DiscIntNeverNeededParam
  Discrete-Time Integrator2 : DiscreteIntegrator  SampleTime=-1  ICPrevOutput=DiscIntNeverNeededParam  ICPrevScaledInput=DiscIntNeverNeededParam
  Divide : Product  Inputs=/*
  Divide2 : Product  Inputs=*/
  Divide3 : Product  Inputs=**///
  Gain1 : Gain  Gain=3
  Gain2 : Gain  Gain=r
  Gain3 : Gain  Gain=b1
  Gain4 : Gain  Gain=b2
  Product{,1..3} (4 alike) : Product
  Scope5 : Scope
  Sign : Signum
  smc_c : Gain  Gain=c
  iq : Outport
  id : Outport  Port=2
  wires:
  uq/1 -> Delay/1
  Delay/1 -> Add2/1
  udc_fbk/1 -> Product3/2, Product3/1
  Product3/1 -> Add/2, [smc_udc_fbk], Add5/1
  udc_ref/1 -> Product2/1, Product2/2
  Product2/1 -> Add/1
  Constant3/1 -> id/1
  [smc_udc_fbk] -> Divide3/1
  Product/1 -> Add3/2
  Gain2/1 -> Add3/1
  Constant4/1 -> Product/2
  Divide3/1 -> Add6/1
  Add3/1 -> Product1/1, Add6/2
  Add6/1 -> iq/1
  Divide2/1 -> Add3/3
  Constant2/1 -> Divide3/5
  [smc_cap] -> Divide3/4
  [b0] -> Divide3/3
  Constant1/1 -> Divide3/2
  Constant/1 -> Add2/2
  Discrete-Time Integrator2/1 -> Gain4/1
  Gain3/1 -> Add4/3
  Add5/1 -> Discrete-Time Integrator2/1, Gain3/1
  Discrete-Time Integrator1/1 -> Add5/2
  Add4/1 -> Discrete-Time Integrator1/1
  Product1/1 -> Add4/2
  [b0] -> Product1/2
  Gain4/1 -> Divide2/1, Add4/1
  [b0] -> Divide2/2
  Sign/1 -> Product/1
  Add1/1 -> Sign/1, Gain2/1
  Divide/1 -> [b0], Scope5/1
  Data Store Read1/1 -> Divide/1, [smc_cap]
  Gain1/1 -> Divide/2
  Add2/1 -> Gain1/1
  Discrete-Time Integrator/1 -> Add1/2
  smc_c/1 -> Discrete-Time Integrator/1
  Add/1 -> Add1/1, smc_c/1

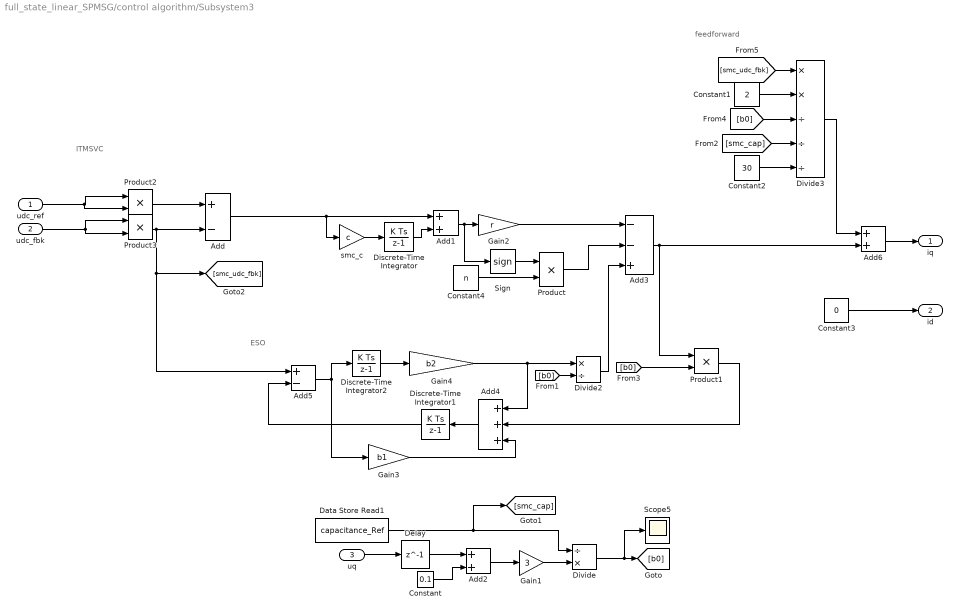
== system full_state_linear_SPMSG/control algorithm/Subsystem3 ==
  note: ITMSVC
  note: feedforward
  note: ESO
  udc_ref : Inport
  udc_fbk : Inport  Port=2
  uq : Inport  Port=3
  Add : Sum  Inputs=+-
  Add1 : Sum
  Add2 : Sum
  Add3 : Sum  Inputs=--+
  Add4 : Sum  Inputs=+++
  Add5 : Sum  Inputs=+-
  Add6 : Sum
  Constant : Constant  Value=0.1  SampleTime=-1
  Constant1 : Constant  Value=2  SampleTime=-1
  Constant2 : Constant  Value=30  SampleTime=-1
  Constant3 : Constant  Value=0  SampleTime=-1
  Constant4 : Constant  Value=n  SampleTime=-1
  Data Store Read1 : DataStoreRead  DataStoreName=capacitance_Ref
  Delay : Delay  DelayLength=1
  Discrete-Time Integrator : DiscreteIntegrator  SampleTime=-1  ICPrevOutput=DiscIntNeverNeededParam  ICPrevScaledInput=DiscIntNeverNeededParam
  Discrete-Time Integrator1 : DiscreteIntegrator  InitialCondition=2304  SampleTime=-1  ICPrevOutput=DiscIntNeverNeededParam  ICPrevScaledInput=DiscIntNeverNeededParam
  Discrete-Time Integrator2 : DiscreteIntegrator  SampleTime=-1  ICPrevOutput=DiscIntNeverNeededParam  ICPrevScaledInput=DiscIntNeverNeededParam
  Divide : Product  Inputs=/*
  Divide2 : Product  Inputs=*/
  Divide3 : Product  Inputs=**///
  Gain1 : Gain  Gain=3
  Gain2 : Gain  Gain=r
  Gain3 : Gain  Gain=b1
  Gain4 : Gain  Gain=b2
  Product{,1..3} (4 alike) : Product
  Scope5 : Scope
  Sign : Signum
  smc_c : Gain  Gain=c
  iq : Outport
  id : Outport  Port=2
  wires:
  Add/1 -> smc_c/1, Add1/1
  smc_c/1 -> Discrete-Time Integrator/1
  Discrete-Time Integrator/1 -> Add1/2
  Add2/1 -> Gain1/1
  Gain1/1 -> Divide/2
  Data Store Read1/1 -> [smc_cap], Divide/1
  Divide/1 -> Scope5/1, [b0]
  Add1/1 -> Gain2/1, Sign/1
  Sign/1 -> Product/1
  [b0] -> Divide2/2
  Gain4/1 -> Add4/1, Divide2/1
  [b0] -> Product1/2
  Product1/1 -> Add4/2
  Add4/1 -> Discrete-Time Integrator1/1
  Discrete-Time Integrator1/1 -> Add5/2
  Add5/1 -> Gain3/1, Discrete-Time Integrator2/1
  Gain3/1 -> Add4/3
  Discrete-Time Integrator2/1 -> Gain4/1
  Constant/1 -> Add2/2
  Constant1/1 -> Divide3/2
  [b0] -> Divide3/3
  [smc_cap] -> Divide3/4
  Constant2/1 -> Divide3/5
  Divide2/1 -> Add3/3
  Add6/1 -> iq/1
  Add3/1 -> Add6/2, Product1/1
  Divide3/1 -> Add6/1
  Constant4/1 -> Product/2
  Gain2/1 -> Add3/1
  Product/1 -> Add3/2
  [smc_udc_fbk] -> Divide3/1
  Constant3/1 -> id/1
  Product2/1 -> Add/1
  udc_ref/1 -> Product2/2, Product2/1
  Product3/1 -> Add5/1, [smc_udc_fbk], Add/2
  udc_fbk/1 -> Product3/1, Product3/2
  Delay/1 -> Add2/1
  uq/1 -> Delay/1

== system full_state_linear_SPMSG/control algorithm/voltage filter ==
  VDCFbk : Inport
  Add : Sum
  Add1 : Sum  Inputs=+-
  Constant : Constant  Value=1000  SampleTime=-1
  Constant1 : Constant  SampleTime=-1
  Delay : Delay  DelayLength=1
  Gain : Gain  Gain=2*pi*TsimCurLoop
  Gain1 : Gain  Gain=2*pi*TsimCurLoop
  Product : Product
  Product1 : Product
  Out1 : Outport
  wires:
  Constant/1 -> Gain1/1, Gain/1
  Gain/1 -> Product/2
  VDCFbk/1 -> Product/1
  Product/1 -> Add/1
  Add/1 -> Delay/1, Out1/1
  Delay/1 -> Product1/1
  Constant1/1 -> Add1/1
  Add1/1 -> Product1/2
  Gain1/1 -> Add1/2
  Product1/1 -> Add/2

== system full_state_linear_SPMSG/control algorithm/voltage filter1 ==
  VDCFbk : Inport
  Add : Sum
  Add1 : Sum  Inputs=+-
  Constant : Constant  Value=0.1  SampleTime=-1
  Constant1 : Constant  SampleTime=-1
  Delay : Delay  DelayLength=1
  Product : Product
  Product1 : Product
  Out1 : Outport
  wires:
  Constant/1 -> Add1/2, Product/2
  VDCFbk/1 -> Product/1
  Product/1 -> Add/1
  Constant1/1 -> Add1/1
  Add1/1 -> Product1/2
  Product1/1 -> Add/2
  [last] -> Delay/1
  Add/1 -> [last], Out1/1
  Delay/1 -> Product1/1

== system full_state_linear_SPMSG/motor/Clark Transformation ==
  U : Inport
  V : Inport  Port=2
  W : Inport  Port=3
  Add : Sum  Inputs=+--
  Add1 : Sum  Inputs=+-
  Gain : Gain  Gain=0.5
  Gain1 : Gain  Gain=0.5
  Gain2 : Gain  Gain=2/3
  Gain3 : Gain  Gain=2/3*0.86602540
  Alpha : Outport
  Beta : Outport  Port=2
  wires:
  V/1 -> Add1/1, Gain/1
  Gain/1 -> Add/2
  W/1 -> Add1/2, Gain1/1
  Gain1/1 -> Add/3
  U/1 -> Add/1
  Add/1 -> Gain2/1
  Gain2/1 -> Alpha/1
  Add1/1 -> Gain3/1
  Gain3/1 -> Beta/1

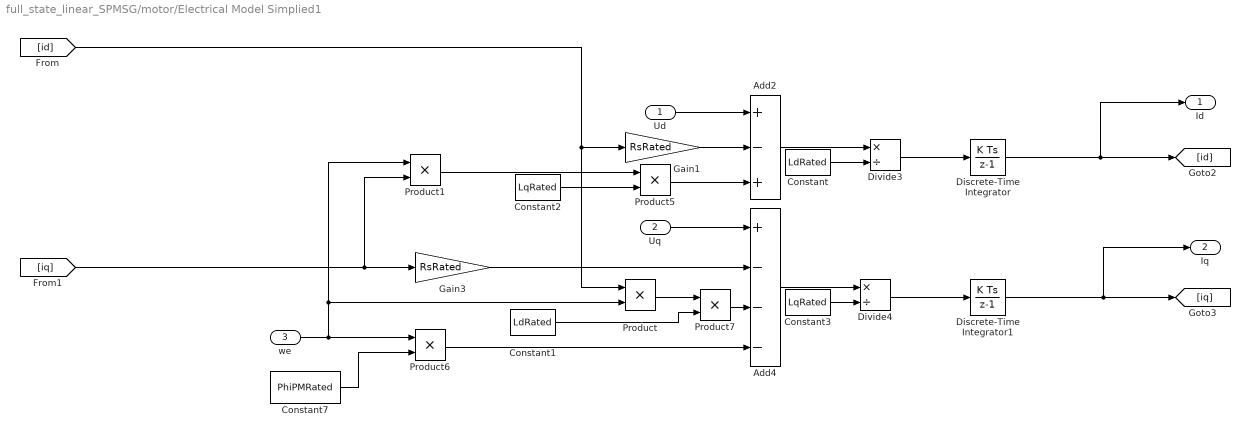
== system full_state_linear_SPMSG/motor/Electrical Model Simplied1 ==
  Ud : Inport
  Uq : Inport  Port=2
  we : Inport  Port=3
  Add2 : Sum  Inputs=+-+
  Add4 : Sum  Inputs=+---
  Constant : Constant  Value=LdRated  SampleTime=TsimMotor
  Constant1 : Constant  Value=LdRated  SampleTime=TsimMotor
  Constant2 : Constant  Value=LqRated  SampleTime=TsimMotor
  Constant3 : Constant  Value=LqRated  SampleTime=TsimMotor
  Constant7 : Constant  Value=PhiPMRated  SampleTime=TsimMotor
  Discrete-Time Integrator : DiscreteIntegrator  SampleTime=TsimMotor  ICPrevOutput=DiscIntNeverNeededParam  ICPrevScaledInput=DiscIntNeverNeededParam
  Discrete-Time Integrator1 : DiscreteIntegrator  SampleTime=TsimMotor  ICPrevOutput=DiscIntNeverNeededParam  ICPrevScaledInput=DiscIntNeverNeededParam
  Divide3 : Product  Inputs=*/
  Divide4 : Product  Inputs=*/
  Gain1 : Gain  Gain=RsRated
  Gain3 : Gain  Gain=RsRated
  Product{,1,5..7} (5 alike) : Product
  Id : Outport
  Iq : Outport  Port=2
  wires:
  Product/1 -> Product7/1
  Discrete-Time Integrator1/1 -> Iq/1, [iq]
  Product5/1 -> Add2/3
  Gain3/1 -> Add4/2
  Product6/1 -> Add4/4
  Discrete-Time Integrator/1 -> Id/1, [id]
  Product7/1 -> Add4/3
  Gain1/1 -> Add2/2
  Add4/1 -> Divide4/1
  Add2/1 -> Divide3/1
  Constant1/1 -> Product7/2
  Divide4/1 -> Discrete-Time Integrator1/1
  Divide3/1 -> Discrete-Time Integrator/1
  [id] -> Product/1, Gain1/1
  [iq] -> Product1/2, Gain3/1
  Ud/1 -> Add2/1
  Uq/1 -> Add4/1
  we/1 -> Product/2, Product1/1, Product6/1
  Constant2/1 -> Product5/2
  Constant/1 -> Divide3/2
  Constant3/1 -> Divide4/2
  Product1/1 -> Product5/1
  Constant7/1 -> Product6/2

== system full_state_linear_SPMSG/motor/Mechanical Model  ==
  speed : Inport
  Discrete-Time Integrator3 : DiscreteIntegrator  SampleTime=TsimMotor  ICPrevOutput=DiscIntNeverNeededParam  ICPrevScaledInput=DiscIntNeverNeededParam
  Gain5 : Gain  Gain=pi*Pn/30
  Theta_e : Outport
  we : Outport  Port=2
  wires:
  Discrete-Time Integrator3/1 -> [theta_e], Theta_e/1
  Gain5/1 -> we/1, Discrete-Time Integrator3/1
  speed/1 -> Gain5/1

== system full_state_linear_SPMSG/motor/Park Transformation ==
  Alpha : Inport
  Beta : Inport  Port=2
  theta : Inport  Port=3
  Add : Sum
  Add1 : Sum  Inputs=+-
  Product{,1..3} (4 alike) : Product
  Sin : Trigonometry  OutputSignalType=real
  Sin1 : Trigonometry  Operator=cos  OutputSignalType=real
  D : Outport
  Q : Outport  Port=2
  wires:
  Product/1 -> Add/1
  Sin/1 -> Product3/2, Product1/2
  Product1/1 -> Add/2
  Add1/1 -> Q/1
  Sin1/1 -> Product2/2, Product/2
  Product2/1 -> Add1/1
  Alpha/1 -> Product3/1, Product/1
  Beta/1 -> Product2/1, Product1/1
  Product3/1 -> Add1/2
  Add/1 -> D/1
  theta/1 -> Sin/1, Sin1/1

== system full_state_linear_SPMSG/motor/VSINonlinearity ==
  IABC : Inport
  Constant : Constant  Value=0.17  SampleTime=TsimMotor
  Constant1 : Constant  SampleTime=TsimMotor
  Demux1 : Demux  Outputs=3
  MATLAB Function1 : MATLAB Function  TreatAsAtomicUnit=on
  MATLAB Function2 : MATLAB Function  TreatAsAtomicUnit=on
  MATLAB Function3 : MATLAB Function  TreatAsAtomicUnit=on
  Mux1 : Mux  Inputs=3
  Scope : Scope
  UError : Outport
  wires:
  Demux1/3 -> MATLAB Function3/1(I)
  Constant1/1 -> MATLAB Function3/3(Vdead), MATLAB Function2/3(Vdead), MATLAB Function1/3(Vdead)
  Constant/1 -> MATLAB Function3/2(K), MATLAB Function2/2(K), MATLAB Function1/2(K)
  MATLAB Function3/1(U) -> Mux1/3
  Demux1/2 -> MATLAB Function2/1(I)
  MATLAB Function2/1(U) -> Mux1/2
  Demux1/1 -> MATLAB Function1/1(I)
  Mux1/1 -> UError/1
  IABC/1 -> Demux1/1
  MATLAB Function1/1(U) -> Scope/1, Mux1/1

== system full_state_linear_SPMSG/control algorithm/CurrentLoop/PI_Id ==
  Id_Ref : Inport
  Id_Fbk : Inport  Port=2
  Add1 : Sum  Inputs=|+-
  Zero-Order Hold5 : ZeroOrderHold  SampleTime=-1
  id实际值 : Scope  NumInputPorts=2
  Ud_PI : Outport
  wires:
  Zero-Order Hold5/1 -> id实际值/2, Add1/2
  Add1/1 -> Ud_PI/1  "uqref"
  Id_Fbk/1 -> Zero-Order Hold5/1
  Id_Ref/1 -> id实际值/1, Add1/1

== system full_state_linear_SPMSG/control algorithm/CurrentLoop/PI_Iq ==
  In1 : Inport
  In2 : Inport  Port=2
  Add2 : Sum  Inputs=|+-
  Zero-Order Hold1 : ZeroOrderHold  SampleTime=-1
  iq实际值 : Scope  NumInputPorts=2
  uqref : Outport
  wires:
  In1/1 -> iq实际值/1, Add2/1
  Zero-Order Hold1/1 -> iq实际值/2, Add2/2
  In2/1 -> Zero-Order Hold1/1
  Add2/1 -> uqref/1  "uqref"

== system full_state_linear_SPMSG/control algorithm/SVPWM1/Inverse Park Transformation ==
  D : Inport
  Q : Inport  Port=2
  theta : Inport  Port=3
  Product{,1..3} (4 alike) : Product  OutDataTypeStr=Inherit: Same as first input
  Sin : Trigonometry  OutputSignalType=real
  Sin1 : Trigonometry  Operator=cos  OutputSignalType=real
  Sum1 : Sum  Inputs=|++  OutDataTypeStr=Inherit: Same as first input
  Sum2 : Sum  Inputs=|+-  OutDataTypeStr=Inherit: Same as first input
  Alpha : Outport
  Beta : Outport  Port=2
  wires:
  Sin1/1 -> Product2/2, Product/2
  Sin/1 -> Product3/2, Product1/2
  Product3/1 -> Sum1/2
  Sum1/1 -> Beta/1
  D/1 -> Product3/1, Product/1
  Product2/1 -> Sum1/1
  Sum2/1 -> Alpha/1
  Product/1 -> Sum2/1
  Product1/1 -> Sum2/2
  Q/1 -> Product2/1, Product1/1
  theta/1 -> Sin/1, Sin1/1

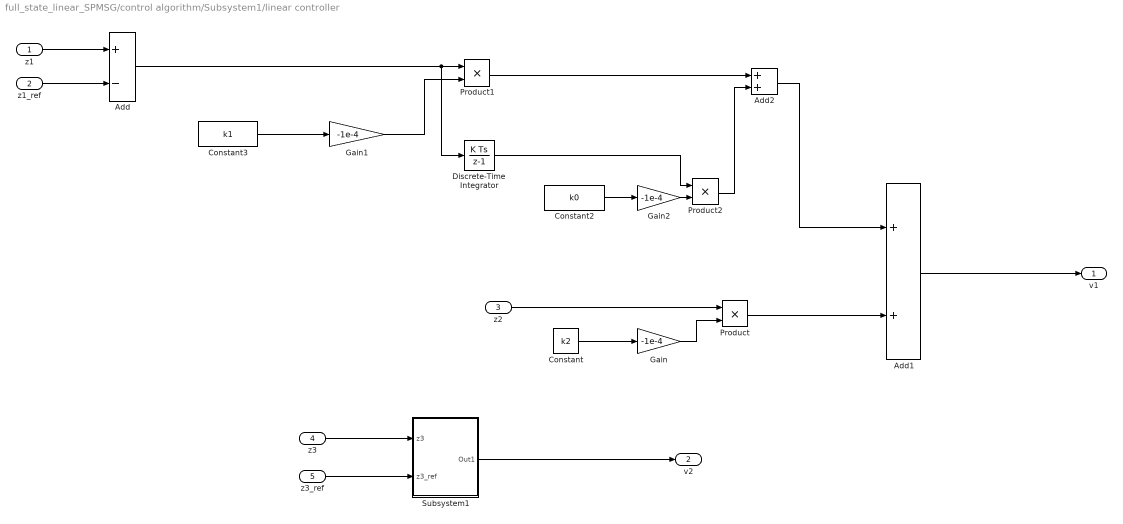
== system full_state_linear_SPMSG/control algorithm/Subsystem1/linear controller ==
  z1 : Inport
  z1_ref : Inport  Port=2
  z2 : Inport  Port=3
  z3 : Inport  Port=4
  z3_ref : Inport  Port=5
  Add : Sum  Inputs=+-
  Add1 : Sum
  Add2 : Sum
  Constant : Constant  Value=k2  SampleTime=-1
  Constant2 : Constant  Value=k0  SampleTime=-1
  Constant3 : Constant  Value=k1  SampleTime=-1
  Discrete-Time Integrator : DiscreteIntegrator  SampleTime=-1  ICPrevOutput=DiscIntNeverNeededParam  ICPrevScaledInput=DiscIntNeverNeededParam
  Gain : Gain  Gain=-1e-4
  Gain1 : Gain  Gain=-1e-4
  Gain2 : Gain  Gain=-1e-4
  Product : Product
  Product1 : Product
  Product2 : Product
  Subsystem1 : Subsystem
  v1 : Outport
  v2 : Outport  Port=2
  wires:
  Constant/1 -> Gain/1
  Gain/1 -> Product/2
  z3/1 -> Subsystem1/1(z3)
  z3_ref/1 -> Subsystem1/2(z3_ref)
  Subsystem1/1(Out1) -> v2/1
  z2/1 -> Product/1
  Product/1 -> Add1/2
  Add2/1 -> Add1/1
  Gain1/1 -> Product1/2
  Gain2/1 -> Product2/2
  z1/1 -> Add/1
  Constant3/1 -> Gain1/1
  z1_ref/1 -> Add/2
  Product1/1 -> Add2/1
  Constant2/1 -> Gain2/1
  Add/1 -> Discrete-Time Integrator/1, Product1/1
  Product2/1 -> Add2/2
  Discrete-Time Integrator/1 -> Product2/1
  Add1/1 -> v1/1

== system full_state_linear_SPMSG/control algorithm/Subsystem1/linear controller/Subsystem1 ==
  z3 : Inport
  z3_ref : Inport  Port=2
  Add : Sum  Inputs=+-
  Add1 : Sum
  Discrete-Time Integrator : DiscreteIntegrator  SampleTime=-1  ICPrevOutput=DiscIntNeverNeededParam  ICPrevScaledInput=DiscIntNeverNeededParam
  Gain : Gain  Gain=-1e-4
  Gain2 : Gain  Gain=-1e-4
  Product : Product
  Product1 : Product
  Subsystem2 : Subsystem  Commented=on
  k3 : Constant  Value=k3  SampleTime=-1
  k4 : Constant  Value=k4  SampleTime=-1
  Out1 : Outport
  wires:
  z3/1 -> Add/1
  z3_ref/1 -> Add/2
  Add/1 -> Product1/1, Product/1
  k3/1 -> Gain/1
  Gain/1 -> Product/2
  Product/1 -> Add1/1
  Add1/1 -> Out1/1
  k4/1 -> Gain2/1
  Product1/1 -> Discrete-Time Integrator/1
  Gain2/1 -> Product1/2
  Discrete-Time Integrator/1 -> Add1/2

== system full_state_linear_SPMSG/control algorithm/Subsystem1/linear controller/Subsystem1/Subsystem2 ==
  In1 : Inport
  In2 : Inport  Port=2
  Add2 : Sum
  Constant : Constant  Value=k4
  Gain : Gain  Gain=TsimCurLoop
  Gain1 : Gain  Gain=-1e-4
  Product : Product
  Out1 : Outport
  wires:
  Gain1/1 -> Gain/1
  Add2/1 -> Out1/1
  Constant/1 -> Gain1/1
  Gain/1 -> Product/1
  In1/1 -> Product/2
  Product/1 -> Add2/1
  In2/1 -> Add2/2

== matlab function full_state_linear_SPMSG/motor/VSINonlinearity/MATLAB Function1 ==
  data: I input; U output; K input; Vdead input
function U = VSI_Nonlinearity(I,K,Vdead)
    U = Vdead*atan(I)/pi*2;
end

== matlab function full_state_linear_SPMSG/motor/VSINonlinearity/MATLAB Function2 ==
  data: I input; U output; K input; Vdead input
function U = VSI_Nonlinearity(I,K,Vdead)
    U = Vdead*atan(I)/pi*2;
end
